simulink model "EEE411L_exp_03"  (R2024b)
settings: Solver=VariableStepAuto  StartTime=0.0  StopTime=10.0  RelTol=1e-3
libraries: simulink x3
settings Model: Creator=fahim  LastModifiedBy=fahim
settings ConfigComp: CovBoundaryAbsTol=1.0e-5

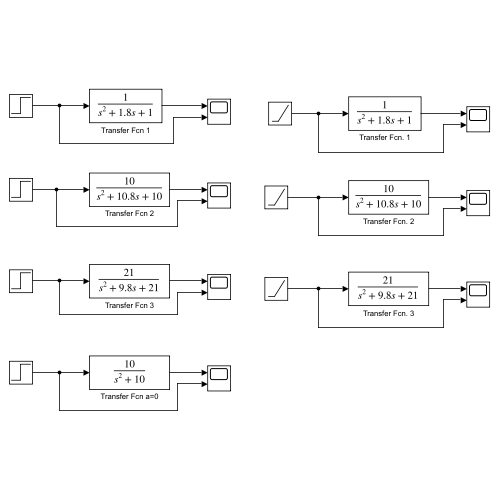
[thumbnail: Simulink's stored preview of the top-level diagram]
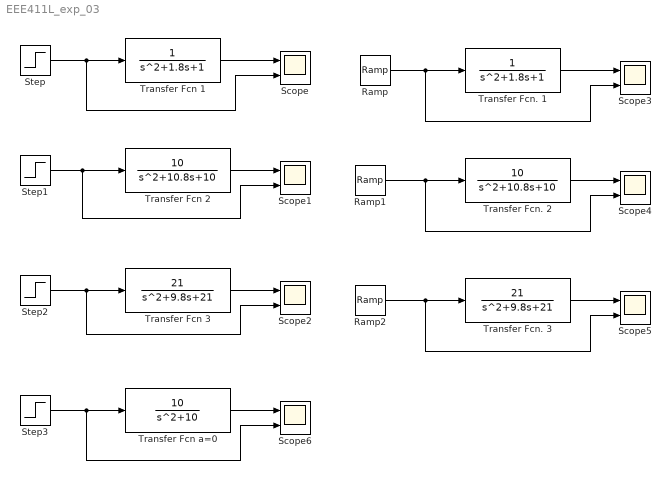
== system EEE411L_exp_03 ==
  Ramp : simulink/Sources/Ramp  slope=1  start=0  InitialOutput=0
  Ramp1 : simulink/Sources/Ramp  slope=1  start=0  InitialOutput=0
  Ramp2 : simulink/Sources/Ramp  slope=1  start=0  InitialOutput=0
  Scope{,1..6} (7 alike) : Scope  NumInputPorts=2
  Step{,1..3} (4 alike) : Step  SampleTime=0
  Transfer Fcn 1 : TransferFcn  Denominator=[1 1.8 1]
  Transfer Fcn 2 : TransferFcn  Numerator=[10]  Denominator=[1 10.8 10]
  Transfer Fcn 3 : TransferFcn  Numerator=[21]  Denominator=[1 9.8 21]
  Transfer Fcn a=0 : TransferFcn  Numerator=[10]  Denominator=[1 0 10]
  Transfer Fcn. 1 : TransferFcn  Denominator=[1 1.8 1]
  Transfer Fcn. 2 : TransferFcn  Numerator=[10]  Denominator=[1 10.8 10]
  Transfer Fcn. 3 : TransferFcn  Numerator=[21]  Denominator=[1 9.8 21]
  wires:
  Transfer Fcn 1/1 -> Scope/1
  Step/1 -> Transfer Fcn 1/1, Scope/2
  Transfer Fcn 2/1 -> Scope1/1
  Step1/1 -> Transfer Fcn 2/1, Scope1/2
  Transfer Fcn 3/1 -> Scope2/1
  Step2/1 -> Transfer Fcn 3/1, Scope2/2
  Transfer Fcn. 2/1 -> Scope4/1
  Transfer Fcn. 1/1 -> Scope3/1
  Ramp2/1 -> Scope5/2, Transfer Fcn. 3/1
  Ramp/1 -> Scope3/2, Transfer Fcn. 1/1
  Transfer Fcn. 3/1 -> Scope5/1
  Ramp1/1 -> Scope4/2, Transfer Fcn. 2/1
  Step3/1 -> Transfer Fcn a=0/1, Scope6/2
  Transfer Fcn a=0/1 -> Scope6/1
